simulink model "Mostar"  (Simulink 10.1)
settings: Solver=FixedStepAuto  StartTime=0  StopTime=7.5  FixedStep=0.005  RelTol=0.001  EnableMultiTasking=on
libraries: fmu_me_lib x2
settings Model: Creator=Tin Rabuzin  LastModifiedBy=meagh
settings DataIOCC: LimitDataPoints=on  OutputSaveName=simout  OutputOption=SpecifiedOutputTimes  OutputTimes=[0:0.005:4.5]
settings OptimizationCC: ExpressionDepthLimit=2147483647
settings DebuggingCC: SolverPrmCheckMsg=warning  StateNameClashWarn=warning
settings GRTTargetCC: CombineOutputUpdateFcns=on  GRTInterface=off

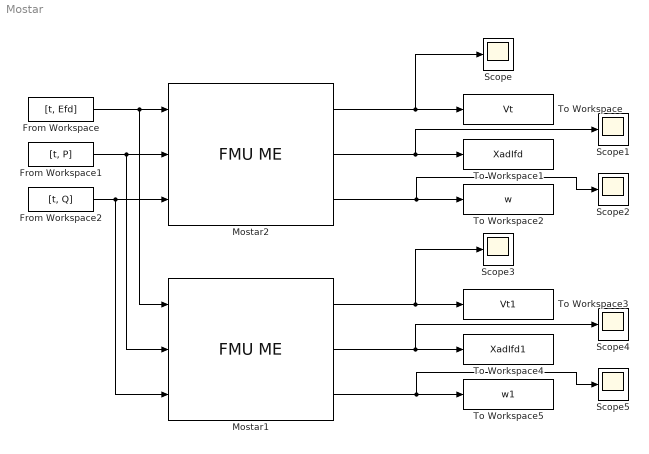
== system Mostar ==
  From Workspace : FromWorkspace  VariableName=[t, Efd]
  From Workspace1 : FromWorkspace  VariableName=[t, P]
  From Workspace2 : FromWorkspace  VariableName=[t, Q]
  Mostar1 : fmu_me_lib/FMU ME  Description=Simulates an FMU for Model Exchange 1.0 or Model Exchange 2.0.  dummy=0
  Mostar2 : fmu_me_lib/FMU ME  Description=Simulates an FMU for Model Exchange 1.0 or Model Exchange 2.0.  dummy=0
  Scope{,1..5} (6 alike) : Scope
  To Workspace : ToWorkspace  VariableName=Vt  SaveFormat=Timeseries  SampleTime=0.005
  To Workspace1 : ToWorkspace  VariableName=XadIfd  SaveFormat=Timeseries  SampleTime=0.005
  To Workspace2 : ToWorkspace  VariableName=w  SaveFormat=Timeseries  SampleTime=0.005
  To Workspace3 : ToWorkspace  VariableName=Vt1  SaveFormat=Timeseries  SampleTime=0.005
  To Workspace4 : ToWorkspace  VariableName=XadIfd1  SaveFormat=Timeseries  SampleTime=0.005
  To Workspace5 : ToWorkspace  VariableName=w1  SaveFormat=Timeseries  SampleTime=0.005
  wires:
  From Workspace/1 -> Mostar1/1, Mostar2/1
  Mostar2/1 -> Scope/1, To Workspace/1
  Mostar2/2 -> Scope1/1, To Workspace1/1
  Mostar2/3 -> Scope2/1, To Workspace2/1
  From Workspace1/1 -> Mostar1/2, Mostar2/2
  From Workspace2/1 -> Mostar1/3, Mostar2/3
  Mostar1/1 -> Scope3/1, To Workspace3/1
  Mostar1/2 -> Scope4/1, To Workspace4/1
  Mostar1/3 -> Scope5/1, To Workspace5/1
